simulink model "AngularFrequency_TestModel"  (R2014a)
settings: Solver=ode45  StartTime=0.0  StopTime=10.0  RelTol=1e-3
libraries: rocket_angular_flight_library x1
settings Model: Creator=scorpii  LastModifiedBy=scorpii

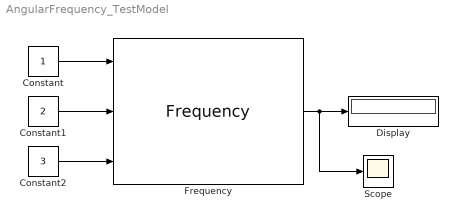
== system AngularFrequency_TestModel ==
  Constant : Constant
  Constant1 : Constant  Value=2
  Constant2 : Constant  Value=3
  Display : Display
  Frequency : rocket_angular_flight_library/Frequency
  Scope : Scope
  wires:
  Constant/1 -> Frequency/1
  Constant1/1 -> Frequency/2
  Constant2/1 -> Frequency/3
  Frequency/1 -> Scope/1, Display/1
